simulink model "sim_controller_A_2015B"  (R2015b)
settings: Solver=VariableStepAuto  StartTime=0.0  StopTime=sim_run  FixedStep=0.001  RelTol=1e-3
InitFcn:
  | zh = 0.01;
undefined symbols (not defined in the file): Standard_Devices, UDP_Protocol, zh_step
libraries: sldrtlib x2, simulink x1
settings Model: Creator=Lenka  LastModifiedBy=Anony
settings DataIOCC: SaveFormat=Array
settings DebuggingCC: SolverPrmCheckMsg=warning
settings HardwareCC: ProdBitPerPointer=32  ProdLargestAtomicFloat=None  ProdIntDivRoundTo=Undefined  ProdEndianess=Unspecified  ProdWordSize=32  ProdHWDeviceType=32-bit Generic
settings GRTTargetCC: GeneratePreprocessorConditionals=Disable all
settings ConfigComp: CovModelRefEnable=Off  CovSFcnEnable=off

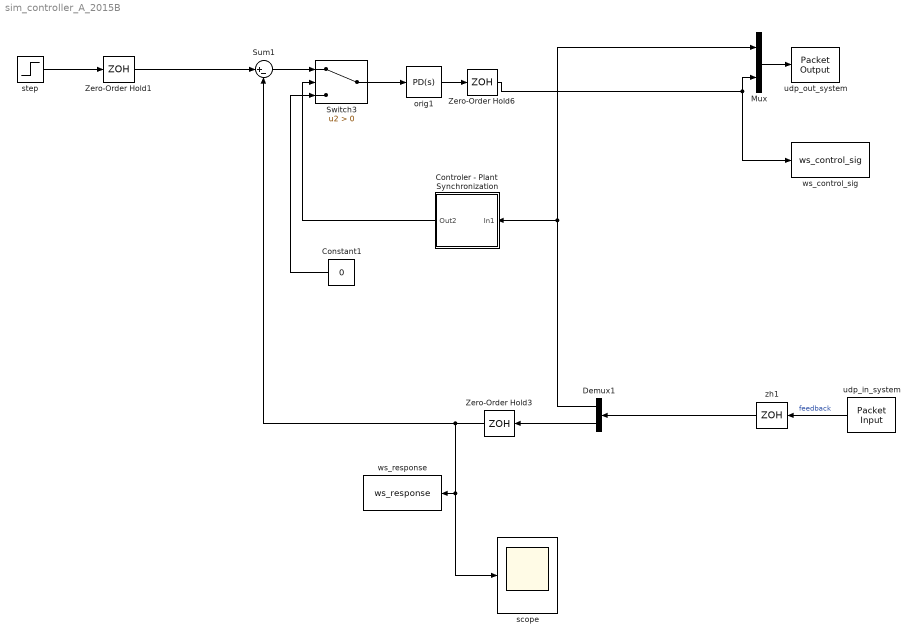
== system sim_controller_A_2015B ==
  Constant1 : Constant  Value=0  SampleTime=zh_step
  Controler - Plant Synchronization : Subsystem
  Demux1 : Demux  Outputs=2
  Mux : Mux  Inputs=2
  Sum1 : Sum  Inputs=|+-
  Switch3 : Switch  Criteria=u2 > Threshold
  Zero-Order Hold1 : ZeroOrderHold  SampleTime=zh_step
  Zero-Order Hold3 : ZeroOrderHold  SampleTime=zh_step
  Zero-Order Hold6 : ZeroOrderHold  SampleTime=zh_step
  orig1 : simulink/Continuous/PID Controller  Controller=PD  TimeDomain=Continuous-time  SampleTime=-1  IntegratorMethod=Forward Euler  FilterMethod=Forward Euler  Form=Parallel  UseFilter=on  ControllerParametersSource=internal  P=0.0142  I=0.0175856984919557  D=0.0001  N=100  InitialConditionSource=internal  InitialConditionForIntegrator=0  InitialConditionForFilter=0  ExternalReset=none  LimitOutput=on  UpperSaturationLimit=5/1000  LowerSaturationLimit=-5/1000  LinearizeAsGain=on  AntiWindupMode=none  Kb=1  TrackingMode=off  Kt=1  PParamMin=[]  PParamMax=[]  IParamMin=[]  IParamMax=[]  DParamMin=[]  DParamMax=[]  NParamMin=[]  NParamMax=[]  KbParamMin=[]  KbParamMax=[]  KtParamMin=[]  KtParamMax=[]  POutMin=[]  POutMax=[]  IOutMin=[]  IOutMax=[]  DOutMin=[]  DOutMax=[]  NOutMin=[]  NOutMax=[]  KbOutMin=[]  KbOutMax=[]  KtOutMin=[]  KtOutMax=[]  IntegratorOutMin=[]  IntegratorOutMax=[]  FilterOutMin=[]  FilterOutMax=[]  SumOutMin=[]  SumOutMax=[]  SumI1OutMin=[]  SumI1OutMax=[]  SumI2OutMin=[]  SumI2OutMax=[]  SumI3OutMin=[]  SumI3OutMax=[]  SumDOutMin=[]  SumDOutMax=[]  SaturationOutMin=[]  SaturationOutMax=[]  IntegratorContinuousStateAttributes=''  IntegratorStateMustResolveToSignalObject=off  IntegratorRTWStateStorageClass=Auto  FilterContinuousStateAttributes=''  FilterStateMustResolveToSignalObject=off  FilterRTWStateStorageClass=Auto  DifferentiatorICPrevScaledInput=0  DifferentiatorOutMin=[]  DifferentiatorOutMax=[]
  scope : Scope
  step : Step  After=0.15  SampleTime=0
  udp_in_system : sldrtlib/Packet Input  SampleTime=0.001  MaxMissedTicks=inf  ShowMissedTicks=off  YieldWhenWaiting=off  DrvName=Standard_Devices/UDP_Protocol  DrvAddress=28500  DrvOptions=[2468394752 28500]  PacketSize=16  DataTypes='2*double'  ShowReady=off  ShowError=off  PacketID=1  ByteOrder=1  ShowTimestamp=off
      settings: AttributesFormatString=Standard Devices\nUDP Protocol [6F54h]
  udp_out_system : sldrtlib/Packet Output  SampleTime=0.01  MaxMissedTicks=inf  ShowMissedTicks=off  YieldWhenWaiting=off  DrvName=Standard_Devices/UDP_Protocol  DrvAddress=27500  DrvOptions=[2468394752 27500]  PacketSize=16  DataTypes='2*double'  ShowReady=off  ShowError=off  PacketID=1  ByteOrder=1  InitialValue=[]  FinalValue=[]
      settings: AttributesFormatString=Standard Devices\nUDP Protocol [6B6Ch]
  ws_control_sig : ToWorkspace  VariableName=ws_control_sig  SaveFormat=Timeseries  SampleTime=zh_step
  ws_response : ToWorkspace  VariableName=ws_response  SaveFormat=Timeseries  SampleTime=zh_step
  zh1 : ZeroOrderHold  SampleTime=zh_step
  wires:
  step/1 -> Zero-Order Hold1/1
  Zero-Order Hold1/1 -> Sum1/1
  orig1/1 -> Zero-Order Hold6/1
  Demux1/2 -> Zero-Order Hold3/1
  Mux/1 -> udp_out_system/1
  Zero-Order Hold6/1 -> Mux/2, ws_control_sig/1
  udp_in_system/1 -> zh1/1  "feedback"
  Zero-Order Hold3/1 -> scope/1, ws_response/1, Sum1/2
  Sum1/1 -> Switch3/1
  Switch3/1 -> orig1/1
  Controler - Plant Synchronization/1(Out2) -> Switch3/2
  Constant1/1 -> Switch3/3
  zh1/1 -> Demux1/1
  Demux1/1 -> Mux/1, Controler - Plant Synchronization/1(In1)

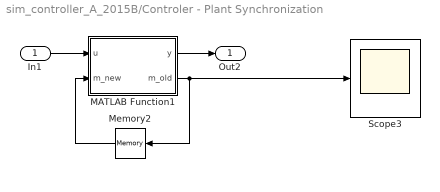
== system sim_controller_A_2015B/Controler - Plant Synchronization ==
  In1 : Inport
  MATLAB Function1 : MATLAB Function  TreatAsAtomicUnit=on
  Memory2 : Memory
  Scope3 : Scope
  Out2 : Outport
  wires:
  MATLAB Function1/2(m_old) -> Memory2/1, Scope3/1
  Memory2/1 -> MATLAB Function1/2(m_new)
  In1/1 -> MATLAB Function1/1(u)
  MATLAB Function1/1(y) -> Out2/1

== matlab function sim_controller_A_2015B/Controler - Plant Synchronization/MATLAB Function1 ==
  data: u input; y output; m_new input; m_old output
function [y, m_old] = fcn(u, m_new)
%#codegen

threshold = 600;

if(u > 0 && m_new < threshold)
    m_old = m_new + 1;
else
    m_old = m_new;
end

if(m_old == threshold)
    y = 1;
else
    y=0;
end
